simulink library "NeoFinansLibrary"  (R2015b)
settings: Solver=ode45  StartTime=0.0  StopTime=10.0  RelTol=1e-3
undefined symbols (not defined in the file or in its folder): Ts
undefined symbols (not defined in the file): car_employees, car_KiEmployeeController, car_KpEmployeeController, car_material, car_price, car_production, car_salary
libraries: simulink x1
settings Model: Creator=ägarenn  LastModifiedBy=Edwin
settings DataIOCC: SaveFormat=Array
settings OptimizationCC: ExpressionDepthLimit=2147483647
settings DebuggingCC: UnderspecifiedInitializationDetection=Classic  MergeDetectMultiDrivingBlocksExec=none  SolverPrmCheckMsg=warning  StateNameClashWarn=warning
settings HardwareCC: ProdBitPerPointer=32  ProdLargestAtomicFloat=None  ProdIntDivRoundTo=Undefined  ProdEndianess=Unspecified  ProdWordSize=32  ProdHWDeviceType=32-bit Generic
settings GRTTargetCC: GeneratePreprocessorConditionals=Disable all
settings ConfigComp: CovModelRefEnable=Off

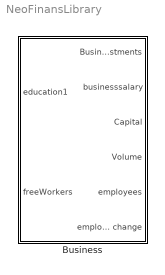
== system NeoFinansLibrary ==
  Business : Subsystem  mask{price=car_price, salary=car_salary, employees=car_employees, effectPerUnit=car_effect_unit, materialCost=car_material, productionCost=car_production, startCapital=10^10, KpEmployeeController=car_KpEmployeeController, KiEmployeeController=car_KiEmployeeController}
      mask prompts: price "Price value"; salary "Salary value"; employees "Number of employees"; effectPerUnit "Effect cost per unit"; materialCost "Material cost"; productionCost "Production cost"; startCapital "Starting Capital"; KpEmployeeController "Kp value in employee contrl."; KiEmployeeController "Ki value in employee contrl."
      mask Display: image(imread('Images/factory.png'))

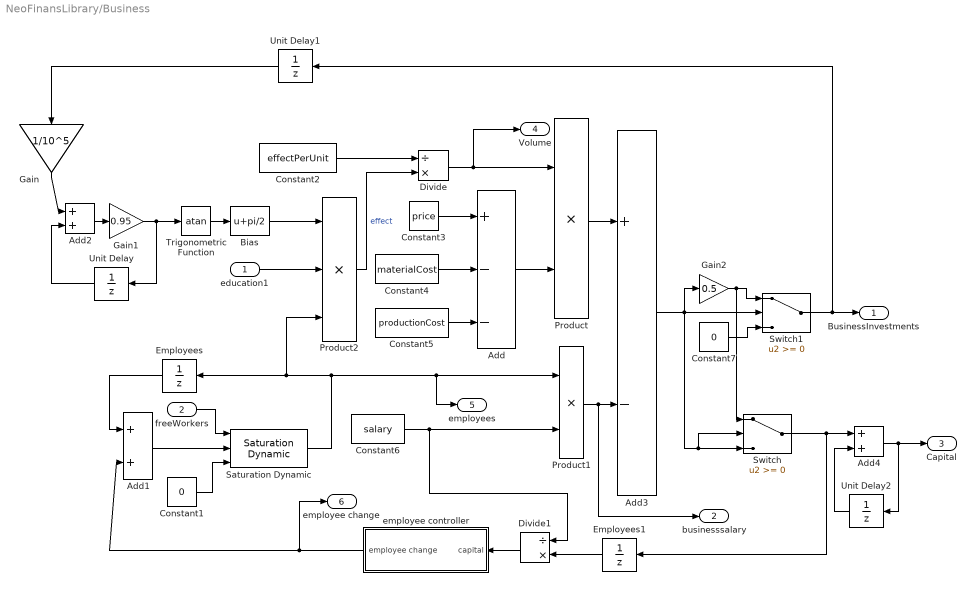
== system NeoFinansLibrary/Business ==
  education1 : Inport
  freeWorkers : Inport  Port=2
  Add : Sum  Inputs=+--
  Add1 : Sum
  Add2 : Sum  Inputs=2
  Add3 : Sum  Inputs=+-
  Add4 : Sum
  Bias : Bias  Bias=pi/2
  Constant1 : Constant  Value=0
  Constant2 : Constant  Value=effectPerUnit
  Constant3 : Constant  Value=price
  Constant4 : Constant  Value=materialCost
  Constant5 : Constant  Value=productionCost
  Constant6 : Constant  Value=salary
  Constant7 : Constant  Value=0
  Divide : Product  Inputs=/*
  Divide1 : Product  Inputs=/*
  Employees : UnitDelay  InitialCondition=employees  SampleTime=-1
  Employees1 : UnitDelay  InitialCondition=startCapital  SampleTime=-1
  Gain : Gain  Gain=1/10^5
  Gain1 : Gain  Gain=0.95
  Gain2 : Gain  Gain=0.5
  Product : Product  RndMeth=Zero
  Product1 : Product  RndMeth=Zero
  Product2 : Product  Inputs=3  RndMeth=Zero
  Saturation Dynamic : simulink/Discontinuities/Saturation Dynamic  OutMin=[]  OutMax=[]  OutDataTypeStr=Inherit: Same as second input  OutDataType=fixdt(1, 16)  OutScaling=2^-10  DoSatur=off
  Switch : Switch
  Switch1 : Switch
  Trigonometric Function : Trigonometry  Operator=atan
  Unit Delay : UnitDelay  InitialCondition=1  SampleTime=-1
  Unit Delay1 : UnitDelay  InitialCondition=1  SampleTime=-1
  Unit Delay2 : UnitDelay  InitialCondition=startCapital  SampleTime=-1
  employee controller : Subsystem
  BusinessInvestments : Outport
  businesssalary : Outport  Port=2
  Capital : Outport  Port=3
  Volume : Outport  Port=4
  employees : Outport  Port=5
  employee change : Outport  Port=6
  wires:
  Constant7/1 -> Switch1/3
  Switch1/1 -> BusinessInvestments/1, Unit Delay1/1
  Add3/1 -> Switch/3, Switch/2, Switch1/2, Gain2/1
  Gain2/1 -> Switch1/1, Switch/1
  Switch/1 -> Add4/1, Employees1/1
  Add4/1 -> Unit Delay2/1, Capital/1
  Unit Delay2/1 -> Add4/2
  Gain1/1 -> Trigonometric Function/1, Unit Delay/1
  Unit Delay1/1 -> Gain/1
  Gain/1 -> Add2/1
  Bias/1 -> Product2/1
  Trigonometric Function/1 -> Bias/1
  Unit Delay/1 -> Add2/2
  Add2/1 -> Gain1/1
  Divide1/1 -> employee controller/1(capital)
  Constant1/1 -> Saturation Dynamic/3
  Add1/1 -> Saturation Dynamic/2
  freeWorkers/1 -> Saturation Dynamic/1
  employee controller/1(employee change) -> employee change/1, Add1/2
  Employees1/1 -> Divide1/2
  Employees/1 -> Add1/1
  Constant2/1 -> Divide/1
  Product1/1 -> businesssalary/1, Add3/2
  education1/1 -> Product2/2
  Divide/1 -> Volume/1, Product/1
  Constant5/1 -> Add/3
  Constant6/1 -> Product1/2, Divide1/1
  Constant3/1 -> Add/1
  Constant4/1 -> Add/2
  Add/1 -> Product/2
  Saturation Dynamic/1 -> Product1/1, employees/1, Product2/3, Employees/1
  Product/1 -> Add3/1
  Product2/1 -> Divide/2  "effect"

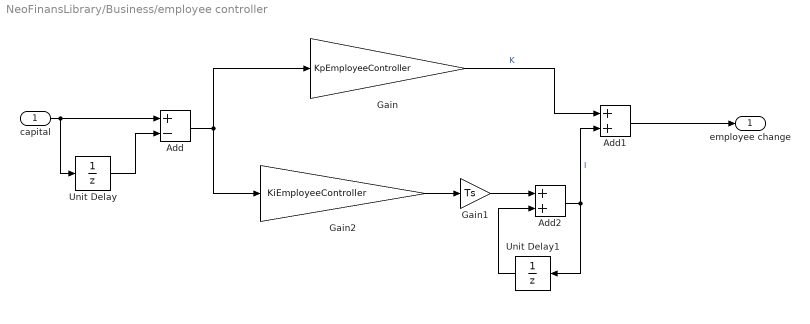
== system NeoFinansLibrary/Business/employee controller ==
  capital : Inport
  Add : Sum  Inputs=+-
  Add1 : Sum
  Add2 : Sum
  Gain : Gain  Gain=KpEmployeeController
  Gain1 : Gain  Gain=Ts
  Gain2 : Gain  Gain=KiEmployeeController
  Unit Delay : UnitDelay  InitialCondition=startCapital/employees  SampleTime=-1
  Unit Delay1 : UnitDelay  SampleTime=-1
  employee change : Outport
  wires:
  Add1/1 -> employee change/1
  capital/1 -> Add/1, Unit Delay/1
  Unit Delay/1 -> Add/2
  Add/1 -> Gain2/1, Gain/1
  Gain/1 -> Add1/1  "K"
  Gain2/1 -> Gain1/1
  Add2/1 -> Unit Delay1/1, Add1/2  "I"
  Gain1/1 -> Add2/1
  Unit Delay1/1 -> Add2/2
